simulink model "09_zvddzvddsspd"  (R2025a)
settings: Solver=FixedStepDiscrete  StartTime=0.0  StopTime=6  FixedStep=Ts  RelTol=1e-3
model workspace (MATLAB code in the model file):
  | N = 11;
  | n = 0:N-1;
  | sigma = (N-1)/6;
  | g = exp(-0.5*((n-(N-1)/2)/sigma).^2);
  | h = g / sum(g);
undefined symbols (not defined in the file): DiscIntNeverNeededParam, Ts
settings Model: Creator=wattanakhonvipanna  LastModifiedBy=wattanakhonvipanna

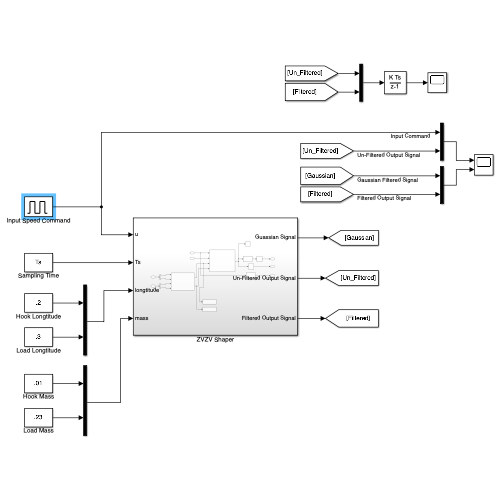
[thumbnail: Simulink's stored preview of the top-level diagram]
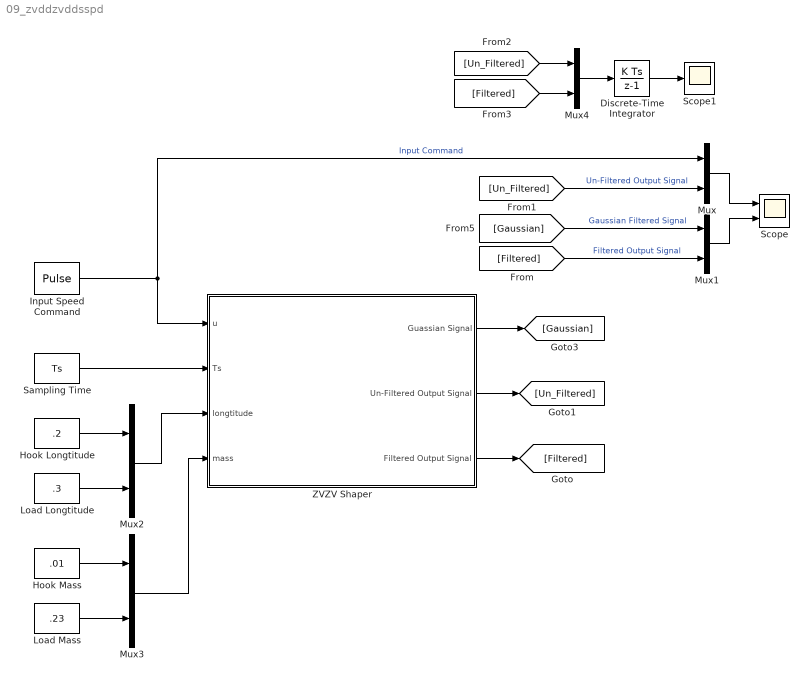
== system 09_zvddzvddsspd ==
  Discrete-Time Integrator : DiscreteIntegrator  SampleTime=-1  ICPrevOutput=DiscIntNeverNeededParam  ICPrevScaledInput=DiscIntNeverNeededParam
  Hook Longtitude : Constant  Value=.2
  Hook Mass : Constant  Value=.01
  Input Speed Command : DiscretePulseGenerator  PulseType=Time based  Amplitude=0.28  Period=6  PulseWidth=50
  Load Longtitude : Constant  Value=.3
  Load Mass : Constant  Value=.23
  Mux{,1..4} (5 alike) : Mux  Inputs=2
  Sampling Time : Constant  Value=Ts
  Scope : Scope  NumInputPorts=2
      settings: ActiveDisplayYMinimum=-0.033375000000000057  ActiveDisplayYMaximum=0.30037499999999995  YLabel=speed (ms^-^1)
  Scope1 : Scope
      settings: ActiveDisplayYMinimum=-0.10012500000000145  ActiveDisplayYMaximum=0.90112500000001328  YLabel=position (m)  DataLoggingVariableName=ScopeData2
  ZVZV Shaper : Subsystem
  wires:
  Sampling Time/1 -> ZVZV Shaper/2(Ts)
  ZVZV Shaper/3(Filtered Output Signal) -> [Filtered]
  ZVZV Shaper/2(Un-Filtered Output Signal) -> [Un_Filtered]
  [Un_Filtered] -> Mux/2  "Un-Filtered Output Signal"
  Mux/1 -> Scope/1
  Input Speed Command/1 -> ZVZV Shaper/1(u), Mux/1  "Input Command"
  Mux1/1 -> Scope/2
  [Gaussian] -> Mux1/1  "Gaussian Filtered Signal"
  [Filtered] -> Mux1/2  "Filtered Output Signal"
  ZVZV Shaper/1(Guassian Signal) -> [Gaussian]
  Mux2/1 -> ZVZV Shaper/3(longtitude)
  Hook Longtitude/1 -> Mux2/1
  Load Longtitude/1 -> Mux2/2
  Load Mass/1 -> Mux3/2
  Hook Mass/1 -> Mux3/1
  Mux3/1 -> ZVZV Shaper/4(mass)
  Mux4/1 -> Discrete-Time Integrator/1
  [Un_Filtered] -> Mux4/1
  [Filtered] -> Mux4/2
  Discrete-Time Integrator/1 -> Scope1/1

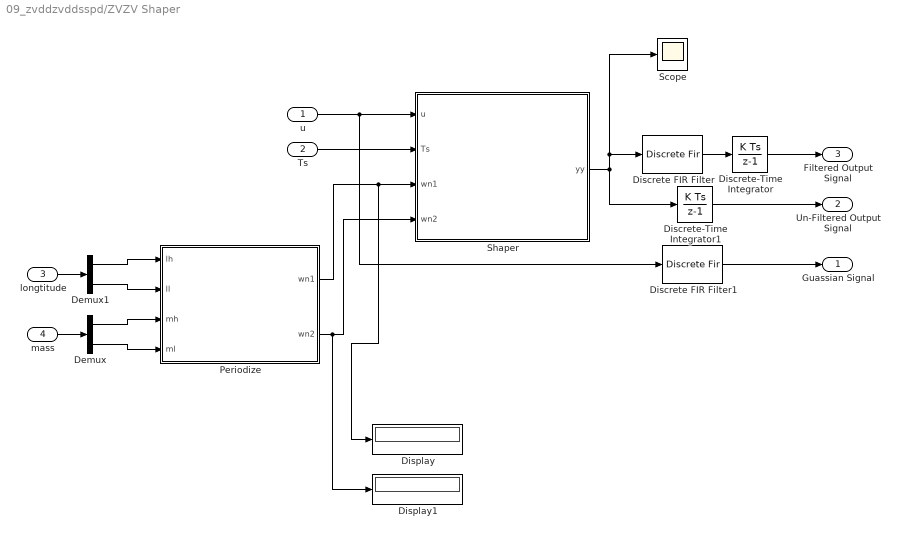
== system 09_zvddzvddsspd/ZVZV Shaper ==
  u : Inport
  Ts : Inport  Port=2
  longtitude : Inport  Port=3
  mass : Inport  Port=4
  Demux : Demux  Outputs=2
  Demux1 : Demux  Outputs=2
  Discrete FIR Filter : DiscreteFir  Coefficients=h
  Discrete FIR Filter1 : DiscreteFir  Coefficients=h
  Discrete-Time Integrator : DiscreteIntegrator  SampleTime=Ts  ICPrevOutput=DiscIntNeverNeededParam  ICPrevScaledInput=DiscIntNeverNeededParam
  Discrete-Time Integrator1 : DiscreteIntegrator  SampleTime=Ts  ICPrevOutput=DiscIntNeverNeededParam  ICPrevScaledInput=DiscIntNeverNeededParam
  Display : Display
  Display1 : Display
  Periodize : MATLAB Function  TreatAsAtomicUnit=on
  Scope : Scope
      settings: ActiveDisplayYMinimum=-9993.7500000000018  ActiveDisplayYMaximum=9993.7500000000018  YLabel=Shaper Impulse (ms^-^2)
  Shaper : MATLAB Function  TreatAsAtomicUnit=on
  Guassian Signal : Outport
  Un-Filtered Output Signal : Outport  Port=2
  Filtered Output Signal : Outport  Port=3
  wires:
  u/1 -> Discrete FIR Filter1/1, Shaper/1(u)
  Ts/1 -> Shaper/2(Ts)
  Discrete-Time Integrator/1 -> Filtered Output Signal/1
  Shaper/1(yy) -> Discrete-Time Integrator1/1, Scope/1, Discrete FIR Filter/1
  Discrete FIR Filter/1 -> Discrete-Time Integrator/1
  Discrete-Time Integrator1/1 -> Un-Filtered Output Signal/1
  Discrete FIR Filter1/1 -> Guassian Signal/1
  mass/1 -> Demux/1
  longtitude/1 -> Demux1/1
  Demux1/1 -> Periodize/1(lh)
  Demux1/2 -> Periodize/2(ll)
  Demux/1 -> Periodize/3(mh)
  Demux/2 -> Periodize/4(ml)
  Periodize/1(wn1) -> Display/1, Shaper/3(wn1)
  Periodize/2(wn2) -> Display1/1, Shaper/4(wn2)

== matlab function 09_zvddzvddsspd/ZVZV Shaper/Periodize ==
  data: lh input; ll input; mh input; wn1 output; wn2 output; ml input
function [wn1, wn2]= ModePeriodize(lh, ll, mh, ml)

g = 9.81;

a = mh * lh * ll;
b = (mh * g * ll) + (ml * g * ll) + (mh * g * lh) + (ml * g * lh);
c = (mh * g * g) + (ml * g * g);

wn1 = sqrt((b - sqrt(b * b - 4 * a * c))/ (2 * a));
wn2 = sqrt((b + sqrt(b * b - 4 * a * c))/ (2 * a));

== matlab function 09_zvddzvddsspd/ZVZV Shaper/Shaper ==
  data: u input; yy output; Ts input; wn1 input; wn2 input
function yy = ZVZVshaper(u, Ts, wn1, wn2)

persistent armed k last_u A_tot d2 d3 d4 d5 d6 d7 d8 d9 d10 d11 d12 d13 ...
    d14 d15 d16
if isempty(armed)
    armed  = false;
    k      = double(0);
    last_u = 0.0;
    A_tot  = 0.0;
    d2     = double(0);
    d3     = double(0);
    d4     = double(0);
    d5     = double(0);
    d6     = double(0);
    d7     = double(0);
    d8     = double(0);
    d9     = double(0);
    d10    = double(0);
    d11    = double(0);
    d12    = double(0);
    d13    = double(0);
    d14    = double(0);
    d15    = double(0);
    d16    = double(0);

end

yy = 0.0;                
tol = 1e-12;

du = u - last_u;
last_u = u;

if ~armed && (abs(du) > tol)
    A_tot = du;
    k     = double(0);
    T1    = 2*pi / max(wn1, 1e-9);
    T2    = 2*pi / max(wn2, 1e-9);
    d2    = double( round( (0.5*T2) / max(Ts,1e-12) ) ); 
    d3    = double( round( T2 / max(Ts,1e-12) ) );
    d4    = double( round( (1.5*T2) / max(Ts,1e-12) ) );
    d5    = double( round( (0.5*T1) / max(Ts,1e-12) ) );
    d6    = double( round( 0.5*(T1+T2) / max(Ts,1e-12) ) );
    d7    = double( round( (0.5*T1+T2) / max(Ts,1e-12) ) );
    d8    = double( round( T1 / max(Ts,1e-12) ) );
    d9    = double( round( (T1+0.5*T2) / max(Ts,1e-12) ) );
    d10   = double( round( (T1+T2) / max(Ts,1e-12) ) );
    d11   = double( round( (T1+1.5*T2) / max(Ts,1e-12) ) );
    d12   = double( round( (1.5*T1) / max(Ts,1e-12) ) );
    d13   = double( round( (1.5*T1+0.5*T2) / max(Ts,1e-12) ) );
    d14   = double( round( (1.5*T1+T2) / max(Ts,1e-12) ) );
    d15   = double( round( (1.5*T1+T2) / max(Ts,1e-12) ) );
    d16   = double( round( (1.5*T1+1.5*T2) / max(Ts,1e-12) ) );
    armed = true;
end


if armed
    if k == double(0)
        yy = ((1/64)*A_tot)  / max(Ts,1e-12);
    elseif k == d2
        yy = ((3/64)*A_tot)  / max(Ts,1e-12);
    elseif k == d3
        yy = ((3/64)*A_tot)  / max(Ts,1e-12);
    elseif k == d4
        yy = ((1/64)*A_tot)  / max(Ts,1e-12);
    elseif k == d5
        yy = ((3/64)*A_tot)  / max(Ts,1e-12);
    elseif k == d6
        yy = ((9/64)*A_tot)  / max(Ts,1e-12);
    elseif k == d7
        yy = ((9/64)*A_tot)  / max(Ts,1e-12);
    elseif k == d8
        yy = ((3/64)*A_tot)  / max(Ts,1e-12);
    elseif k == d9
        yy = ((3/64)*A_tot)  / max(Ts,1e-12);
    elseif k == d10
        yy = ((9/64)*A_tot)  / max(Ts,1e-12);
    elseif k == d11
        yy = ((9/64)*A_tot)  / max(Ts,1e-12);
    elseif k == d12
        yy = ((3/64)*A_tot)  / max(Ts,1e-12);
    elseif k == d13
        yy = ((1/64)*A_tot)  / max(Ts,1e-12);
    elseif k == d14
        yy = ((3/64)*A_tot)  / max(Ts,1e-12);
    elseif k == d15
        yy = ((3/64)*A_tot)  / max(Ts,1e-12);
    elseif k == d16
        yy = ((1/64)*A_tot)  / max(Ts,1e-12);
    end

    k = k + double(1);
    if k > d16 + double(1)
        armed = false;
    end
end
